simulink model "Dynamics_EquationsOfMotion_TH"  (Simulink 7.8)
settings: Solver=ode45  StartTime=0.0  StopTime=10  RelTol=1e-3
libraries: AeroSim x1
settings Model: Creator=Ryan  LastModifiedBy=Ryan

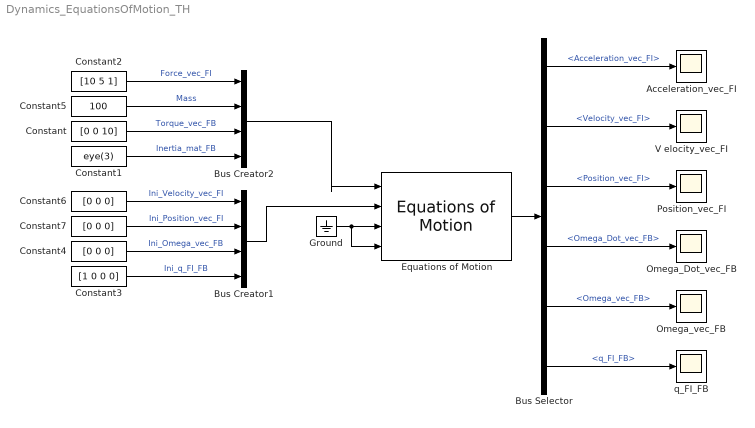
== system Dynamics_EquationsOfMotion_TH ==
  Acceleration_vec_FI : Scope
      settings: SaveName=ScopeData3
  Bus Creator1 : BusCreator
  Bus Creator2 : BusCreator
  Bus Selector : BusSelector  OutputSignals=Acceleration_vec_FI,Velocity_vec_FI,Position_vec_FI,Omega_Dot_vec_FB,Omega_vec_FB,q_FI_FB
  Constant : Constant  Value=[0 0 10]
  Constant1 : Constant  Value=eye(3)
  Constant2 : Constant  Value=[10 5 1]
  Constant3 : Constant  Value=[1 0 0 0]
  Constant4 : Constant  Value=[0 0 0]
  Constant5 : Constant  Value=100
  Constant6 : Constant  Value=[0 0 0]
  Constant7 : Constant  Value=[0 0 0]
  Equations of Motion : AeroSim/Dynamics/Equations of Motion
  Ground : Ground
  Omega_Dot_vec_FB : Scope
  Omega_vec_FB : Scope
  Position_vec_FI : Scope
      settings: SaveName=ScopeData4
  V elocity_vec_FI : Scope
      settings: SaveName=ScopeData5
  q_FI_FB : Scope
      settings: SaveName=ScopeData2
  wires:
  Ground/1 -> Equations of Motion/4, Equations of Motion/3
  Bus Creator2/1 -> Equations of Motion/1
  Bus Creator1/1 -> Equations of Motion/2
  Equations of Motion/1 -> Bus Selector/1
  Bus Selector/4 -> Omega_Dot_vec_FB/1  "<Omega_Dot_vec_FB>"
  Bus Selector/5 -> Omega_vec_FB/1  "<Omega_vec_FB>"
  Bus Selector/6 -> q_FI_FB/1  "<q_FI_FB>"
  Constant4/1 -> Bus Creator1/3  "Ini_Omega_vec_FB"
  Constant3/1 -> Bus Creator1/4  "Ini_q_FI_FB"
  Constant5/1 -> Bus Creator2/2  "Mass"
  Constant2/1 -> Bus Creator2/1  "Force_vec_FI"
  Constant7/1 -> Bus Creator1/2  "Ini_Position_vec_FI"
  Constant6/1 -> Bus Creator1/1  "Ini_Velocity_vec_FI"
  Constant1/1 -> Bus Creator2/4  "Inertia_mat_FB"
  Constant/1 -> Bus Creator2/3  "Torque_vec_FB"
  Bus Selector/1 -> Acceleration_vec_FI/1  "<Acceleration_vec_FI>"
  Bus Selector/2 -> V elocity_vec_FI/1  "<Velocity_vec_FI>"
  Bus Selector/3 -> Position_vec_FI/1  "<Position_vec_FI>"
